simulink model "Observer"  (R2021b)
settings: Solver=VariableStepAuto  StartTime=0.0  StopTime=10.0  RelTol=1e-3
libraries: aerolibutil x2
settings Model: Creator=jorgemarrero  LastModifiedBy=jorgemarrero

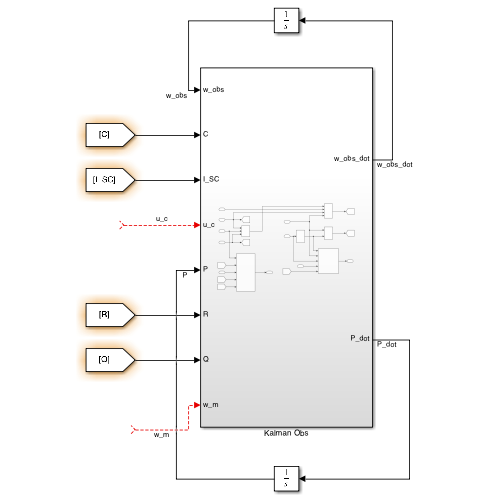
[thumbnail: Simulink's stored preview of the top-level diagram]
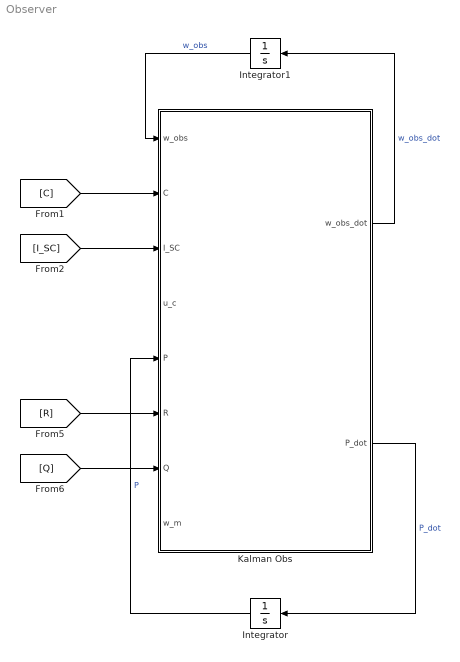
== system Observer ==
  Integrator : Integrator
  Integrator1 : Integrator
  Kalman Obs : Subsystem
  wires:
  [C] -> Kalman Obs/2(C)
  [I_SC] -> Kalman Obs/3(I_SC)
  ? -> Kalman Obs/4(u_c)  "u_c"
  [R] -> Kalman Obs/6(R)
  [Q] -> Kalman Obs/7(Q)
  ? -> Kalman Obs/8(w_m)  "w_m"
  Kalman Obs/2(P_dot) -> Integrator/1  "P_dot"
  Integrator/1 -> Kalman Obs/5(P)  "P"
  Kalman Obs/1(w_obs_dot) -> Integrator1/1  "w_obs_dot"
  Integrator1/1 -> Kalman Obs/1(w_obs)  "w_obs"

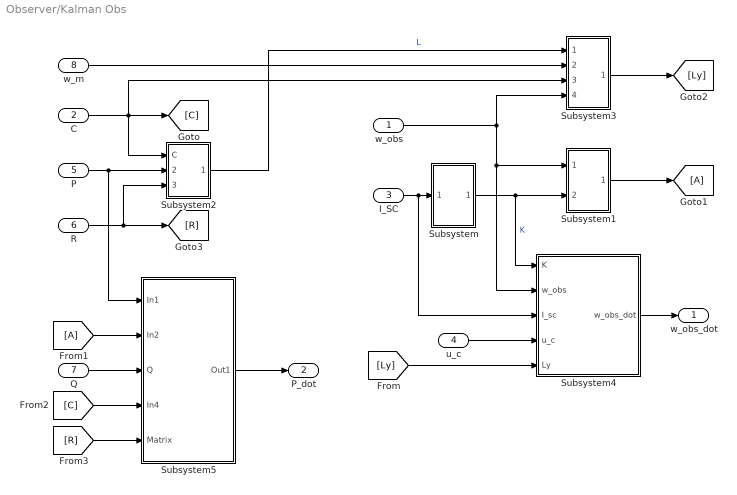
== system Observer/Kalman Obs ==
  w_obs : Inport
  C : Inport  Port=2
  I_SC : Inport  Port=3
  u_c : Inport  Port=4
  P : Inport  Port=5
  R : Inport  Port=6
  Q : Inport  Port=7
  w_m : Inport  Port=8
  Subsystem : Subsystem
  Subsystem1 : Subsystem
  Subsystem2 : Subsystem
  Subsystem3 : Subsystem
  Subsystem4 : Subsystem
  Subsystem5 : Subsystem
  w_obs_dot : Outport
  P_dot : Outport  Port=2
  wires:
  I_SC/1 -> Subsystem4/3(I_sc), Subsystem/1(In1)
  Subsystem/1(Out1) -> Subsystem4/1(K), Subsystem1/2(In2)  "K"
  w_obs/1 -> Subsystem4/2(w_obs), Subsystem1/1(In1), Subsystem3/4(In4)
  Subsystem1/1(Out1) -> [A]
  C/1 -> Subsystem3/3(In3), [C], Subsystem2/1(C)
  P/1 -> Subsystem5/1(In1), Subsystem2/2(In2)
  R/1 -> Subsystem2/3(Matrix), [R]
  Subsystem2/1(Out1) -> Subsystem3/1(In1)  "L"
  w_m/1 -> Subsystem3/2(In2)
  Subsystem3/1(Out1) -> [Ly]
  Subsystem4/1(w_obs_dot) -> w_obs_dot/1
  u_c/1 -> Subsystem4/4(u_c)
  [Ly] -> Subsystem4/5(Ly)
  [A] -> Subsystem5/2(In2)
  Q/1 -> Subsystem5/3(Q)
  [C] -> Subsystem5/4(In4)
  [R] -> Subsystem5/5(Matrix)
  Subsystem5/1(Out1) -> P_dot/1

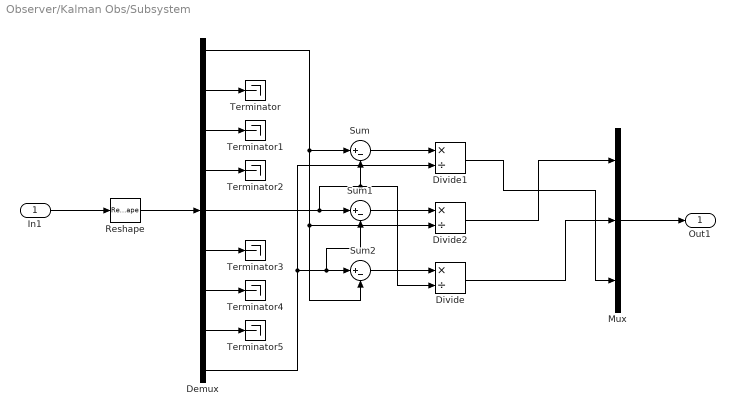
== system Observer/Kalman Obs/Subsystem ==
  In1 : Inport
  Demux : Demux  Outputs=9
  Divide : Product  Inputs=*/
  Divide1 : Product  Inputs=*/
  Divide2 : Product  Inputs=*/
  Mux : Mux  Inputs=3
  Reshape : Reshape  OutputDimensionality=Column vector (2-D)
  Sum : Sum  Inputs=|+-
  Sum1 : Sum  Inputs=|+-
  Sum2 : Sum  Inputs=|+-
  Terminator{,1..5} (6 alike) : Terminator
  Out1 : Outport
  wires:
  Mux/1 -> Out1/1
  Divide2/1 -> Mux/1
  Sum2/1 -> Divide/1
  Divide1/1 -> Mux/3
  Sum/1 -> Divide1/1
  Demux/1 -> Sum2/2, Divide2/2, Sum/1
  Sum1/1 -> Divide2/1
  Divide/1 -> Mux/2
  Demux/9 -> Divide1/2, Sum1/2, Sum2/1
  Demux/5 -> Divide/2, Sum/2, Sum1/1
  In1/1 -> Reshape/1
  Reshape/1 -> Demux/1
  Demux/2 -> Terminator/1
  Demux/3 -> Terminator1/1
  Demux/4 -> Terminator2/1
  Demux/6 -> Terminator3/1
  Demux/7 -> Terminator4/1
  Demux/8 -> Terminator5/1

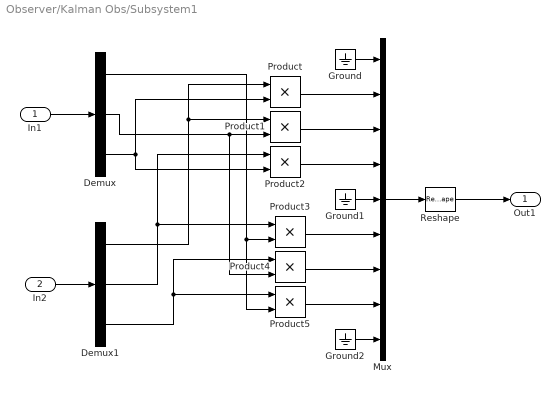
== system Observer/Kalman Obs/Subsystem1 ==
  In1 : Inport
  In2 : Inport  Port=2
  Demux : Demux  Outputs=3
  Demux1 : Demux  Outputs=3
  Ground : Ground
  Ground1 : Ground
  Ground2 : Ground
  Mux : Mux  Inputs=9
  Product{,1..5} (6 alike) : Product
  Reshape : Reshape  OutputDimensionality=Customize  OutputDimensions=[3,3]
  Out1 : Outport
  wires:
  Reshape/1 -> Out1/1
  Mux/1 -> Reshape/1
  Demux/3 -> Product2/2, Product/2
  Product3/1 -> Mux/6
  Product4/1 -> Mux/7
  In1/1 -> Demux/1
  Demux1/1 -> Product1/1, Product/1
  Product5/1 -> Mux/8
  Ground2/1 -> Mux/9
  Demux1/3 -> Product5/1, Product4/1
  Product1/1 -> Mux/3
  Ground/1 -> Mux/1
  Product/1 -> Mux/2
  Product2/1 -> Mux/4
  In2/1 -> Demux1/1
  Demux/2 -> Product4/2, Product1/2
  Demux1/2 -> Product2/1, Product3/1
  Ground1/1 -> Mux/5
  Demux/1 -> Product5/2, Product3/2

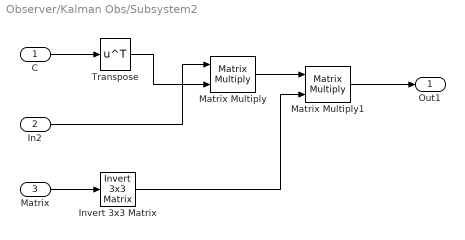
== system Observer/Kalman Obs/Subsystem2 ==
  C : Inport
  In2 : Inport  Port=2
  Matrix : Inport  Port=3
  Invert 3x3 Matrix : aerolibutil/Invert  3x3 Matrix
  Matrix Multiply : Product  Multiplication=Matrix(*)
  Matrix Multiply1 : Product  Multiplication=Matrix(*)
  Transpose : Math  Operator=transpose  SaturateOnIntegerOverflow=on
  Out1 : Outport
  wires:
  Matrix Multiply1/1 -> Out1/1
  In2/1 -> Matrix Multiply/1
  Transpose/1 -> Matrix Multiply/2
  C/1 -> Transpose/1
  Matrix Multiply/1 -> Matrix Multiply1/1
  Matrix/1 -> Invert 3x3 Matrix/1
  Invert 3x3 Matrix/1 -> Matrix Multiply1/2

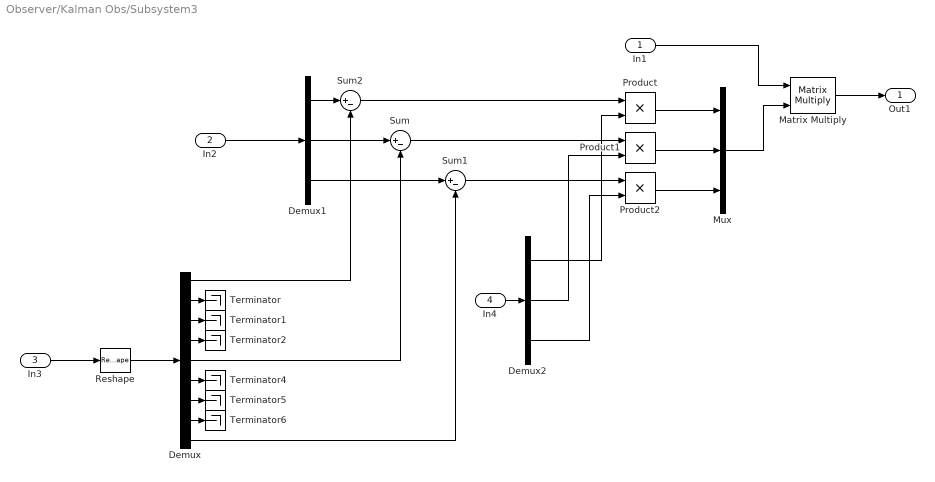
== system Observer/Kalman Obs/Subsystem3 ==
  In1 : Inport
  In2 : Inport  Port=2
  In3 : Inport  Port=3
  In4 : Inport  Port=4
  Demux : Demux  Outputs=9
  Demux1 : Demux  Outputs=3
  Demux2 : Demux  Outputs=3
  Matrix Multiply : Product  Multiplication=Matrix(*)
  Mux : Mux  Inputs=3
  Product : Product
  Product1 : Product
  Product2 : Product
  Reshape : Reshape  OutputDimensionality=Column vector (2-D)
  Sum : Sum  Inputs=|+-
  Sum1 : Sum  Inputs=|+-
  Sum2 : Sum  Inputs=|+-
  Terminator{,1..2,4..6} (6 alike) : Terminator
  Out1 : Outport
  wires:
  In4/1 -> Demux2/1
  Matrix Multiply/1 -> Out1/1
  In2/1 -> Demux1/1
  Demux/3 -> Terminator1/1
  Product2/1 -> Mux/3
  Product1/1 -> Mux/2
  Demux/1 -> Sum2/2
  Demux1/1 -> Sum2/1
  Demux/4 -> Terminator2/1
  Demux/2 -> Terminator/1
  Demux1/2 -> Sum/1
  Demux2/2 -> Product1/2
  Demux1/3 -> Sum1/1
  In1/1 -> Matrix Multiply/1
  Mux/1 -> Matrix Multiply/2
  Demux2/1 -> Product/2
  Demux/8 -> Terminator6/1
  Sum1/1 -> Product2/1
  Demux/5 -> Sum/2
  Sum/1 -> Product1/1
  Demux/7 -> Terminator5/1
  Demux2/3 -> Product2/2
  Product/1 -> Mux/1
  Demux/9 -> Sum1/2
  Demux/6 -> Terminator4/1
  Reshape/1 -> Demux/1
  Sum2/1 -> Product/1
  In3/1 -> Reshape/1

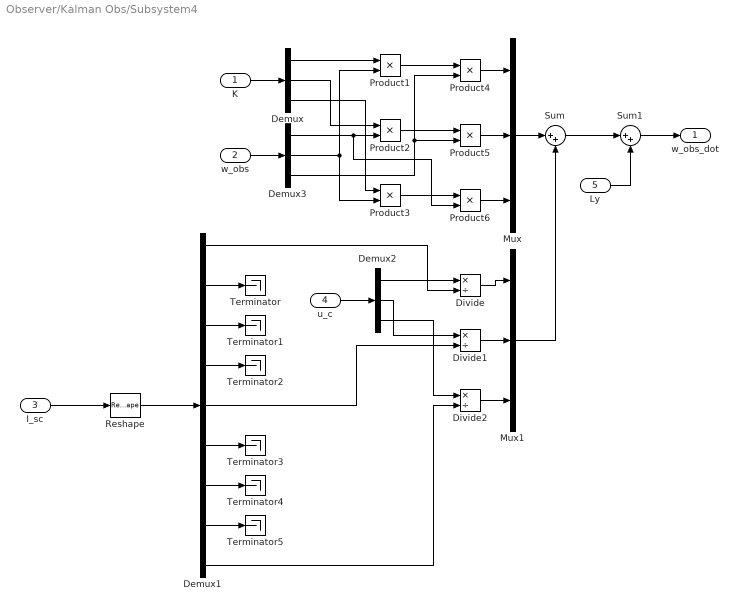
== system Observer/Kalman Obs/Subsystem4 ==
  K : Inport
  w_obs : Inport  Port=2
  I_sc : Inport  Port=3
  u_c : Inport  Port=4
  Ly : Inport  Port=5
  Demux : Demux  Outputs=3
  Demux1 : Demux  Outputs=9
  Demux2 : Demux  Outputs=3
  Demux3 : Demux  Outputs=3
  Divide : Product  Inputs=*/
  Divide1 : Product  Inputs=*/
  Divide2 : Product  Inputs=*/
  Mux : Mux  Inputs=3
  Mux1 : Mux  Inputs=3
  Product{1..6} (6 alike) : Product
  Reshape : Reshape  OutputDimensionality=Column vector (2-D)
  Sum : Sum  Inputs=|++
  Sum1 : Sum  Inputs=|++
  Terminator{,1..5} (6 alike) : Terminator
  w_obs_dot : Outport
  wires:
  K/1 -> Demux/1
  u_c/1 -> Demux2/1
  w_obs/1 -> Demux3/1
  Ly/1 -> Sum1/2
  Demux/1 -> Product1/1
  Demux3/2 -> Product3/2, Product1/2
  Demux/2 -> Product2/1
  Demux/3 -> Product3/1
  Demux3/1 -> Product6/2, Product2/2
  Product1/1 -> Product4/1
  Product2/1 -> Product5/1
  Product3/1 -> Product6/1
  Demux3/3 -> Product5/2, Product4/2
  Demux2/1 -> Divide/1
  Demux2/2 -> Divide1/1
  Demux2/3 -> Divide2/1
  Demux1/1 -> Divide/2
  Demux1/5 -> Divide1/2
  Demux1/9 -> Divide2/2
  Product5/1 -> Mux/2
  Product4/1 -> Mux/1
  Product6/1 -> Mux/3
  Divide/1 -> Mux1/1
  Divide1/1 -> Mux1/2
  Divide2/1 -> Mux1/3
  Mux/1 -> Sum/1
  Mux1/1 -> Sum/2
  Sum/1 -> Sum1/1
  Sum1/1 -> w_obs_dot/1
  Demux1/3 -> Terminator1/1
  Demux1/7 -> Terminator4/1
  Reshape/1 -> Demux1/1
  I_sc/1 -> Reshape/1
  Demux1/6 -> Terminator3/1
  Demux1/2 -> Terminator/1
  Demux1/8 -> Terminator5/1
  Demux1/4 -> Terminator2/1

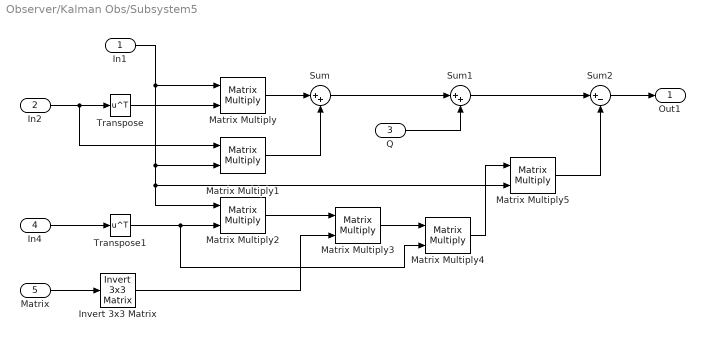
== system Observer/Kalman Obs/Subsystem5 ==
  In1 : Inport
  In2 : Inport  Port=2
  Q : Inport  Port=3
  In4 : Inport  Port=4
  Matrix : Inport  Port=5
  Invert 3x3 Matrix : aerolibutil/Invert  3x3 Matrix
  Matrix Multiply{,1..5} (6 alike) : Product  Multiplication=Matrix(*)
  Sum : Sum  Inputs=|++
  Sum1 : Sum  Inputs=|++
  Sum2 : Sum  Inputs=|+-
  Transpose : Math  Operator=transpose  SaturateOnIntegerOverflow=on
  Transpose1 : Math  Operator=transpose  SaturateOnIntegerOverflow=on
  Out1 : Outport
  wires:
  In4/1 -> Transpose1/1
  Matrix Multiply2/1 -> Matrix Multiply3/1
  Sum1/1 -> Sum2/1
  Transpose/1 -> Matrix Multiply/2
  Transpose1/1 -> Matrix Multiply4/2, Matrix Multiply2/2
  Matrix/1 -> Invert 3x3 Matrix/1
  Matrix Multiply3/1 -> Matrix Multiply4/1
  Q/1 -> Sum1/2
  Matrix Multiply1/1 -> Sum/2
  Matrix Multiply4/1 -> Matrix Multiply5/1
  Matrix Multiply/1 -> Sum/1
  Matrix Multiply5/1 -> Sum2/2
  Sum/1 -> Sum1/1
  In2/1 -> Matrix Multiply1/1, Transpose/1
  In1/1 -> Matrix Multiply/1, Matrix Multiply2/1, Matrix Multiply5/2, Matrix Multiply1/2
  Sum2/1 -> Out1/1
  Invert 3x3 Matrix/1 -> Matrix Multiply3/2
